simulink model "FixedwingModelR2020b"  (R2020b)
settings: Solver=ode4  StartTime=0.0  StopTime=100  FixedStep=0.001  RelTol=1e-3
PreLoadFcn:
  | filepath  = fileparts(get_param(bdroot, 'FileName'))
  | cd(filepath);
InitFcn:
  | Init
  | InitData
values from neighbouring files (symbols this model uses):
  env = struct    [InitData.m]
  ModelInit_Inputs = [0 0 -1 0 0 0 0 0 0 0 0 0 0 0 0 0]    [Init.m]
  ModelParam_envAltitude = -50    [Init.m]
  ModelParam_GPSEphFinal = 0.3    [Init.m]
  ModelParam_GPSEpvFinal = 0.4    [Init.m]
  ModelParam_noiseGPSSampTime = 0.2    [Init.m]
  ModelParam_noisePowerOffGainAccel = 0.04    [Init.m]
  ModelParam_noisePowerOffGainAccelZ = 0.03    [Init.m]
  ModelParam_noisePowerOffGainGyro = 0.02    [Init.m]
  ModelParam_noisePowerOffGainGyroZ = 0.025    [Init.m]
  ModelParam_noisePowerOffGainMag = 0.02    [Init.m]
  ModelParam_noisePowerOffGainMagZ = 0.035    [Init.m]
  ModelParam_noisePowerOnGainAccel = 0.8    [Init.m]
  ModelParam_noisePowerOnGainAccelZ = 4.5    [Init.m]
  ModelParam_noisePowerOnGainGyro = 2    [Init.m]
  ModelParam_noisePowerOnGainGyroZ = 1    [Init.m]
  ModelParam_noisePowerOnGainMag = 0.025    [Init.m]
  ModelParam_noisePowerOnGainMagZ = 0.05    [Init.m]
  ModelParam_uavType = int8(100)    [Init.m]
  uav = struct    [InitData.m]
undefined symbols (not defined in the file or in its folder): Earth, F, Light, MIL, ModelParam_GPSEpvInitial, ModelParam_GPSEpvTimeConstant, Newton, Raphson, WGS84
libraries: sharedtransform x6, aerolibactuator x5, FixedwingModelLib x4, aerolibasang x4, aerolibtransform2 x2, aerolibatmos2 x2, aerolibconvert2 x2, simulink x2, aerolibutil x2, aerolibwind2 x2, aerolibobsolete x1, shared6dof x1
(part 1 of 2)
settings Model: Creator=Jinrui  LastModifiedBy=dzl20201126
settings DataIOCC: ReturnWorkspaceOutputs=off
settings OptimizationCC: ZeroExternalMemoryAtStartup=off  ZeroInternalMemoryAtStartup=off  EfficientTunableParamExpr=on
settings DebuggingCC: ParameterTunabilityLossMsg=error  ArithmeticOperatorsInVariantConditions=warning
settings SFSimCC: SimUseLocalCustomCode=off  MATLABDynamicMemAlloc=off  CustomCodeUndefinedFunction=UseInterfaceOnly  SimTargetLang=C++
settings RTWCC: Description=Embedded Coder  SystemTargetFile=ert.tlc  GenCodeOnly=on  GenerateMakefile=off  PackageGeneratedCodeAndArtifacts=on  PackageName=MulticopterModel  TemplateMakefile=ert_default_tmf  RTWUseLocalCustomCode=off  TargetLang=C++  RTWCompilerOptimization=on
settings CodeAppCC: ForceParamTrailComments=on  OperatorAnnotations=on  SimulinkDataObjDesc=on  SFDataObjDesc=on  MATLABFcnDesc=on  InsertBlockDesc=on  StateflowObjectComments=on  MATLABSourceComments=on
settings ERTTargetCC: TargetLangStandard=C++03 (ISO)  MultiwordLength=2048  GenerateSampleERTMain=on  CodeInterfacePackaging=C++ class  SupportContinuousTime=on  MultiInstanceErrorCode=None  RootIOFormat=Structure reference  ERTCustomFileTemplate=example_file_process.tlc  ERTFilePackagingFormat=Compact
settings SimscapeCC: SimscapeNormalizeSystem=off

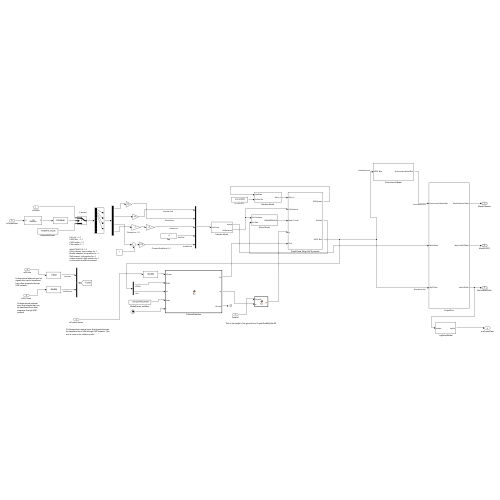
[thumbnail: Simulink's stored preview of the top-level diagram]
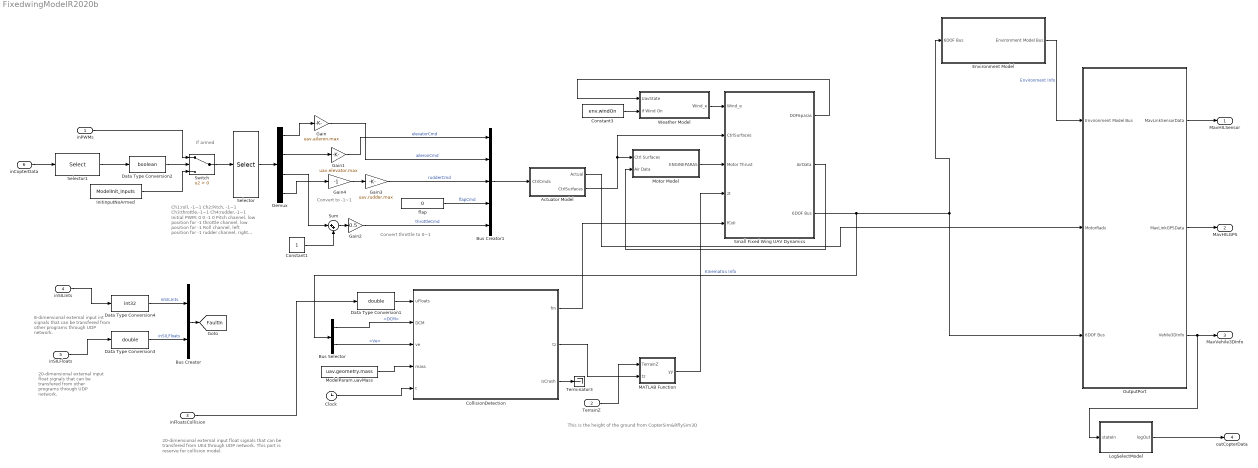
== system FixedwingModelR2020b ==
  note: Convert to -1~1
  note: Convert throttle to 0~1
  note: Ch1:roll, -1~1
      | Ch2:Pitch, -1~1
      | Ch3:throttle,-1~1
      | Ch4:rudder,-1~1
      |
      | Initial PWM: 0 0 -1 0
      | Pitch channel, low position for -1
      | throttle channel, low position for -1
      | Roll channel, left position for -1
      | rudder channel, right position for -1, so the value should be reversed
  note: This is the height of the ground from CopterSim&RflySim3D
  note: 20-dimensional external input float signals that can be transfered from UE4 through UDP network. This port is reserve for collision model.
  note: If armed
  note: 20-dimensional external input float signals that can be transfered from other programs through UDP network.
  note: 8-dimensional external input int signals that can be transfered from other programs through UDP network.
  inPWMs : Inport  PortDimensions=16
  TerrainZ : Inport  Port=2
  inFloatsCollision : Inport  Port=3  OutDataTypeStr=single  PortDimensions=20
  inSILInts : Inport  Port=4  OutDataTypeStr=int32  PortDimensions=8
  inSILFloats : Inport  Port=5  OutDataTypeStr=single  PortDimensions=20
  inCopterData : Inport  Port=6  OutDataTypeStr=double  PortDimensions=32
  Actuator Model : Subsystem
  Bus Creator : BusCreator  Inputs=2
  Bus Creator1 : BusCreator  Inputs=5
  Bus Selector : BusSelector  OutputSignals=DCM,Ve
  Clock : Clock
  CollisionDetection : MATLAB Function  TreatAsAtomicUnit=on
  Constant1 : Constant
  Constant3 : Constant  Value=env.windOn
      settings: AttributesFormatString=%<Value>
  Data Type Conversion1 : DataTypeConversion  OutDataTypeStr=double
  Data Type Conversion2 : DataTypeConversion  OutDataTypeStr=boolean
  Data Type Conversion3 : DataTypeConversion  OutDataTypeStr=double
  Data Type Conversion4 : DataTypeConversion  OutDataTypeStr=int32
  Demux : Demux
  Environment Model : Subsystem
  Gain : Gain  Gain=uav.aileron.max
  Gain1 : Gain  Gain=uav.elevator.max
  Gain2 : Gain  Gain=0.5
  Gain3 : Gain  Gain=uav.rudder.max
  Gain4 : Gain  Gain=-1
  InitinputNoArmed : Constant  Value=ModelInit_Inputs
  LogSelectModel : Subsystem
  MATLAB Function : MATLAB Function  TreatAsAtomicUnit=on
  ModelParam.uavMass : Constant  Value=uav.geometry.mass
  Motor Model : Subsystem
  OutputPort : Subsystem
  Selector : Selector  InputPortWidth=16  IndexOptions=Index vector (dialog)  Indices=[1 2 3 4]  OutputSizes=1
  Selector1 : Selector  InputPortWidth=32  IndexOptions=Index vector (dialog)  Indices=[1]  OutputSizes=1
  Small Fixed Wing UAV Dynamics : Subsystem
  Sum : Sum  Inputs=|++
  Switch : Switch  Criteria=u2 > Threshold
  Terminator3 : Terminator
  Weather Model : Subsystem
  flap : Constant  Value=0  OutDataTypeStr=double
  MavHILSensor : Outport  OutDataTypeStr=Bus: MavLinkSensor  VectorParamsAs1DForOutWhenUnconnected=off
  MavHILGPS : Outport  Port=2  OutDataTypeStr=Bus: MavLinkGPS  VectorParamsAs1DForOutWhenUnconnected=off
  MavVehile3DInfo : Outport  Port=3  OutDataTypeStr=Bus: MavVehileInfo  VectorParamsAs1DForOutWhenUnconnected=off
  outCopterData : Outport  Port=4  OutDataTypeStr=double  PortDimensions=32  VectorParamsAs1DForOutWhenUnconnected=off
  tag scope: FaultIn=global
  wires:
  Sum/1 -> Gain2/1
  Actuator Model/1(Actual) -> OutputPort/2(MotorRads)
  Demux/3 -> Sum/1
  Demux/1 -> Gain/1
  inPWMs/1 -> Switch/1
  Selector/1 -> Demux/1
  Demux/2 -> Gain1/1
  Small Fixed Wing UAV Dynamics/3(6DOF Bus) -> Bus Selector/1, Environment Model/1(6DOF Bus), OutputPort/3(6DOF Bus)  "Kinematics Info"
  Constant1/1 -> Sum/2
  Environment Model/1(Environment Model Bus) -> OutputPort/1(Environment Model Bus)  "Environment Info"
  Switch/1 -> Selector/1
  CollisionDetection/2(tz) -> MATLAB Function/2(tz)
  Actuator Model/2(CtrlSurfaces) -> Motor Model/1(Ctrl Surfaces), Small Fixed Wing UAV Dynamics/2(CtrlSurfaces)
  Small Fixed Wing UAV Dynamics/1(DOF6paras) -> Weather Model/1(UavState)
  Motor Model/1(ENGINEPARAS) -> Small Fixed Wing UAV Dynamics/3(Motor Thrust)
  Bus Creator1/1 -> Actuator Model/1(CtrlCmds)
  Constant3/1 -> Weather Model/2(if Wind On)
  Weather Model/1(Wind_e) -> Small Fixed Wing UAV Dynamics/1(Wind_e)
  Small Fixed Wing UAV Dynamics/2(AirData) -> Motor Model/2(Air Data)
  Gain3/1 -> Bus Creator1/3  "rudderCmd"
  flap/1 -> Bus Creator1/4  "flapCmd"
  Gain/1 -> Bus Creator1/2  "aileronCmd"
  Gain1/1 -> Bus Creator1/1  "elevatorCmd"
  Demux/4 -> Gain4/1
  Gain2/1 -> Bus Creator1/5  "throttleCmd"
  Gain4/1 -> Gain3/1
  CollisionDetection/1(fm) -> Small Fixed Wing UAV Dynamics/5(fColi)
  TerrainZ/1 -> MATLAB Function/1(TerrainZ)
  Bus Selector/1 -> CollisionDetection/2(DCM)  "<DCM>"
  Bus Selector/2 -> CollisionDetection/3(ve)  "<Ve>"
  ModelParam.uavMass/1 -> CollisionDetection/4(mass)
  Clock/1 -> CollisionDetection/5(t)
  Data Type Conversion1/1 -> CollisionDetection/1(uFloats)
  MATLAB Function/1(yy) -> Small Fixed Wing UAV Dynamics/4(zt)
  inFloatsCollision/1 -> Data Type Conversion1/1
  CollisionDetection/3(isCrash) -> Terminator3/1
  OutputPort/3(Vehile3DInfo) -> LogSelectModel/1(stateIn), MavVehile3DInfo/1
  OutputPort/2(MavLinkGPSData) -> MavHILGPS/1
  OutputPort/1(MavLinkSensorData) -> MavHILSensor/1
  Selector1/1 -> Data Type Conversion2/1
  inCopterData/1 -> Selector1/1
  InitinputNoArmed/1 -> Switch/3
  Data Type Conversion2/1 -> Switch/2
  Data Type Conversion3/1 -> Bus Creator/2  "inSILFloats"
  Bus Creator/1 -> [FaultIn]
  inSILFloats/1 -> Data Type Conversion3/1
  inSILInts/1 -> Data Type Conversion4/1
  Data Type Conversion4/1 -> Bus Creator/1  "inSILInts"
  LogSelectModel/1(logOut) -> outCopterData/1

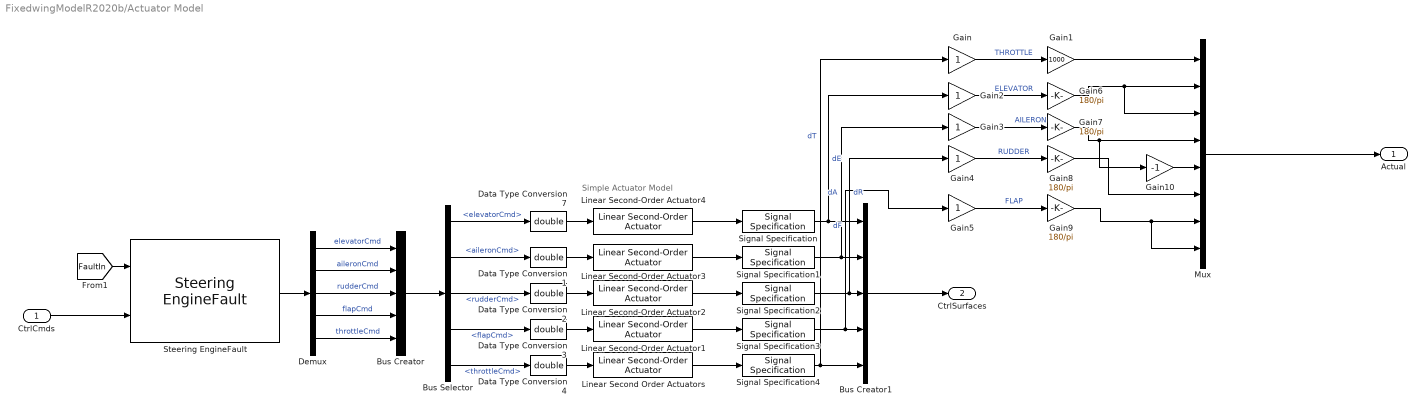
== system FixedwingModelR2020b/Actuator Model ==
  note: Simple Actuator Model
  CtrlCmds : Inport
  Bus Creator : BusCreator  Inputs=5
  Bus Creator1 : BusCreator  Inputs=5
  Bus Selector : BusSelector  OutputSignals=elevatorCmd,aileronCmd,rudderCmd,flapCmd,throttleCmd
  Data Type Conversion{1..4,7} (5 alike) : DataTypeConversion  OutDataTypeStr=double
  Demux : Demux  Outputs=5
  Gain{,2..5} (5 alike) : Gain
  Gain1 : Gain  Gain=1000
  Gain10 : Gain  Gain=-1
  Gain{6..9} (4 alike) : Gain  Gain=180/pi
  Linear Second Order Actuators : aerolibactuator/Linear Second-Order Actuator  wn_fin=35  z_fin=0.75  fin_act_0=0  fin_act_vel=0
      settings: SourceProductBaseCode=AE
      settings: AttributesFormatString=|
      | Nat Freq => %<wn_fin>
      | Damping => %<z_fin>
  Linear Second-Order Actuator{1..4} (4 alike) : aerolibactuator/Linear Second-Order Actuator  wn_fin=35  z_fin=0.75  fin_act_0=0  fin_act_vel=0
      settings: SourceProductBaseCode=AE
  Mux : Mux  Inputs=8
  Signal Specification{,1..3} (4 alike) : SignalSpecification  Unit=rad
  Signal Specification4 : SignalSpecification  Unit=%
  Steering EngineFault : FixedwingModelLib/Steering EngineFault  FaultParamStruct=SteerEngineFault  ComParamVect=FaultParamAPI
  Actual : Outport  VectorParamsAs1DForOutWhenUnconnected=off
  CtrlSurfaces : Outport  Port=2  VectorParamsAs1DForOutWhenUnconnected=off
  wires:
  Data Type Conversion7/1 -> Linear Second-Order Actuator4/1
  Data Type Conversion1/1 -> Linear Second-Order Actuator3/1
  Data Type Conversion2/1 -> Linear Second-Order Actuator2/1
  Data Type Conversion3/1 -> Linear Second-Order Actuator1/1
  Data Type Conversion4/1 -> Linear Second Order Actuators/1
  Bus Selector/1 -> Data Type Conversion7/1  "<elevatorCmd>"
  Linear Second-Order Actuator2/1 -> Signal Specification2/1
  Linear Second-Order Actuator3/1 -> Signal Specification1/1
  Linear Second-Order Actuator1/1 -> Signal Specification3/1
  Linear Second-Order Actuator4/1 -> Signal Specification/1
  Bus Selector/4 -> Data Type Conversion3/1  "<flapCmd>"
  Bus Selector/5 -> Data Type Conversion4/1  "<throttleCmd>"
  Bus Selector/3 -> Data Type Conversion2/1  "<rudderCmd>"
  Bus Selector/2 -> Data Type Conversion1/1  "<aileronCmd>"
  Linear Second Order Actuators/1 -> Signal Specification4/1
  Signal Specification/1 -> Gain2/1, Bus Creator1/1  "dE"
  Signal Specification1/1 -> Gain3/1, Bus Creator1/2  "dA"
  Signal Specification2/1 -> Gain4/1, Bus Creator1/3  "dR"
  Signal Specification4/1 -> Gain/1, Bus Creator1/5  "dT"
  Gain1/1 -> Mux/1
  Gain/1 -> Gain1/1  "THROTTLE"
  Gain2/1 -> Gain6/1  "ELEVATOR"
  Gain4/1 -> Gain8/1  "RUDDER"
  Gain3/1 -> Gain7/1  "AILERON"
  Signal Specification3/1 -> Gain5/1, Bus Creator1/4  "dF"
  Gain5/1 -> Gain9/1  "FLAP"
  Gain6/1 -> Mux/3, Mux/2
  Gain7/1 -> Gain10/1, Mux/4
  Gain8/1 -> Mux/6
  Gain9/1 -> Mux/8, Mux/7
  Gain10/1 -> Mux/5
  Mux/1 -> Actual/1
  Bus Creator1/1 -> CtrlSurfaces/1
  Demux/3 -> Bus Creator/3  "rudderCmd"
  Demux/5 -> Bus Creator/5  "throttleCmd"
  Demux/1 -> Bus Creator/1  "elevatorCmd"
  [FaultIn] -> Steering EngineFault/1
  Demux/4 -> Bus Creator/4  "flapCmd"
  Steering EngineFault/1 -> Demux/1
  Demux/2 -> Bus Creator/2  "aileronCmd"
  CtrlCmds/1 -> Steering EngineFault/2
  Bus Creator/1 -> Bus Selector/1

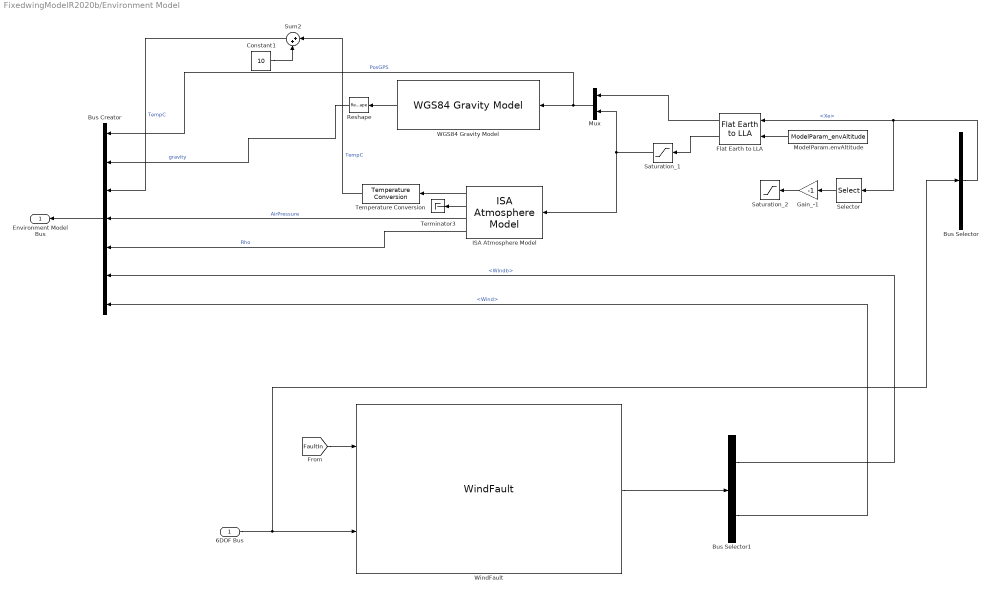
== system FixedwingModelR2020b/Environment Model ==
  6DOF Bus : Inport
  Bus Creator : BusCreator  Inputs=7
  Bus Selector : BusSelector  OutputSignals=Xe
  Bus Selector1 : BusSelector  OutputSignals=Windb,Wind
  Constant1 : Constant  Value=10
  Flat Earth to LLA : aerolibtransform2/Flat Earth to LLA  units=Metric (MKS)  ptype=Earth (WGS84)  F=1/298.257223563  R=6378137  refPosPort=off  LL0=ModelParam_GPSLatLong  psi=0
  Gain_-1 : Gain  Gain=-1
  ISA Atmosphere Model : aerolibatmos2/ISA Atmosphere Model  custom=off  g=9.80665  gamma=1.4  R=287.0531  L=0.0065  h_trop=11000  h_strat=20000  rho0=1.225  P0=101325  T0=288.15  h0=0
  ModelParam.envAltitude : Constant  Value=ModelParam_envAltitude
  Mux : Mux  Inputs=2
  Reshape : Reshape
  Saturation_1 : Saturate  UpperLimit=100000  LowerLimit=0
  Saturation_2 : Saturate  UpperLimit=10000  LowerLimit=0
  Selector : Selector  InputPortWidth=3  IndexOptions=Index vector (dialog)  Indices=[3]  OutputSizes=1
  Sum2 : Sum  Inputs=|++
  Temperature Conversion : aerolibconvert2/Temperature Conversion  IU=K  OU=C
      settings: SourceProductBaseCode=AE
  Terminator3 : Terminator
  "WGS84 Gravity Model " : aerolibobsolete/WGS84 Gravity Model   model=WGS84 Taylor Series  units=Metric (MKS)  no_atmos=on  precessing=on  jd_loc=off  month=October  day=10  year=2004  no_centrifugal=on  action=Warning
      settings: SourceProductBaseCode=AE
  WindFault : FixedwingModelLib/WindFault  FaultParamStruct=WindFault  ComParamVect=FaultParamAPI
  Environment Model Bus : Outport  VectorParamsAs1DForOutWhenUnconnected=off
  wires:
  ISA Atmosphere Model/4 -> Bus Creator/5  "Rho"
  [FaultIn] -> WindFault/1
  6DOF Bus/1 -> WindFault/2, Bus Selector/1
  Flat Earth to LLA/2 -> Saturation_1/1
  WindFault/1 -> Bus Selector1/1
  Sum2/1 -> Bus Creator/3  "TempC"
  ModelParam.envAltitude/1 -> Flat Earth to LLA/2
  Gain_-1/1 -> Saturation_2/1
  Bus Selector1/1 -> Bus Creator/6  "<Windb>"
  Saturation_1/1 -> Mux/2, ISA Atmosphere Model/1
  ISA Atmosphere Model/1 -> Temperature Conversion/1
  "WGS84 Gravity Model "/1 -> Reshape/1
  Bus Selector1/2 -> Bus Creator/7  "<Wind>"
  Bus Creator/1 -> Environment Model Bus/1
  Bus Selector/1 -> Selector/1, Flat Earth to LLA/1  "<Xe>"
  Temperature Conversion/1 -> Sum2/1  "TempC"
  Mux/1 -> Bus Creator/1, "WGS84 Gravity Model "/1  "PosGPS"
  Selector/1 -> Gain_-1/1
  ISA Atmosphere Model/3 -> Bus Creator/4  "AirPressure"
  Flat Earth to LLA/1 -> Mux/1
  ISA Atmosphere Model/2 -> Terminator3/1
  Reshape/1 -> Bus Creator/2  "gravity"
  Constant1/1 -> Sum2/2

== system FixedwingModelR2020b/LogSelectModel ==
  note: 1:3
  note: 4:6
  note: 7:9
  stateIn : Inport
  Bus Selector : BusSelector  OutputSignals=AccB,RateB,VelE
  Bus Selector1 : BusSelector  OutputSignals=PWM
  Constant : Constant  Value=[0,0,0,0,0,0,0,0,0,0,0,0,0,0,0,0,0,0]
  Data Type Conversion{,1..3} (4 alike) : DataTypeConversion  OutDataTypeStr=double
  Mux12 : Mux  Inputs=5
  logOut : Outport
  wires:
  stateIn/1 -> Bus Selector/1
  Bus Selector/1 -> Data Type Conversion/1  "<AccB>"
  Bus Selector/2 -> Data Type Conversion1/1  "<RateB>"
  Bus Selector/3 -> Data Type Conversion2/1  "<VelE>"
  [is123450] -> Bus Selector1/1
  Bus Selector1/1 -> Data Type Conversion3/1  "<PWM>"
  Data Type Conversion/1 -> Mux12/1
  Data Type Conversion1/1 -> Mux12/2
  Data Type Conversion2/1 -> Mux12/3
  Data Type Conversion3/1 -> Mux12/4
  Mux12/1 -> logOut/1
  Constant/1 -> Mux12/5

== system FixedwingModelR2020b/Motor Model ==
  Ctrl Surfaces : Inport
  Air Data : Inport  Port=2
  Bus Creator1 : BusCreator  Inputs=6
  Bus Selector : BusSelector  OutputSignals=dT
  Bus Selector1 : BusSelector  OutputSignals=airpseed
  Constant{1..5} (5 alike) : Constant  Value=0
  Engine Model : Subsystem
  ENGINEPARAS : Outport  VectorParamsAs1DForOutWhenUnconnected=off
  wires:
  Bus Selector1/1 -> Engine Model/2(Airspeed)  "<airpseed>"
  Ctrl Surfaces/1 -> Bus Selector/1
  Air Data/1 -> Bus Selector1/1
  Bus Selector/1 -> Engine Model/1(dt)  "<dT>"
  Engine Model/1(Thrust_b) -> Bus Creator1/1  "Fx_eng"
  Constant4/1 -> Bus Creator1/5  "M_eng"
  Constant3/1 -> Bus Creator1/4  "R_eng"
  Constant5/1 -> Bus Creator1/6  "N_eng"
  Constant2/1 -> Bus Creator1/3  "Fz_eng"
  Constant1/1 -> Bus Creator1/2  "Fy_eng"
  Bus Creator1/1 -> ENGINEPARAS/1

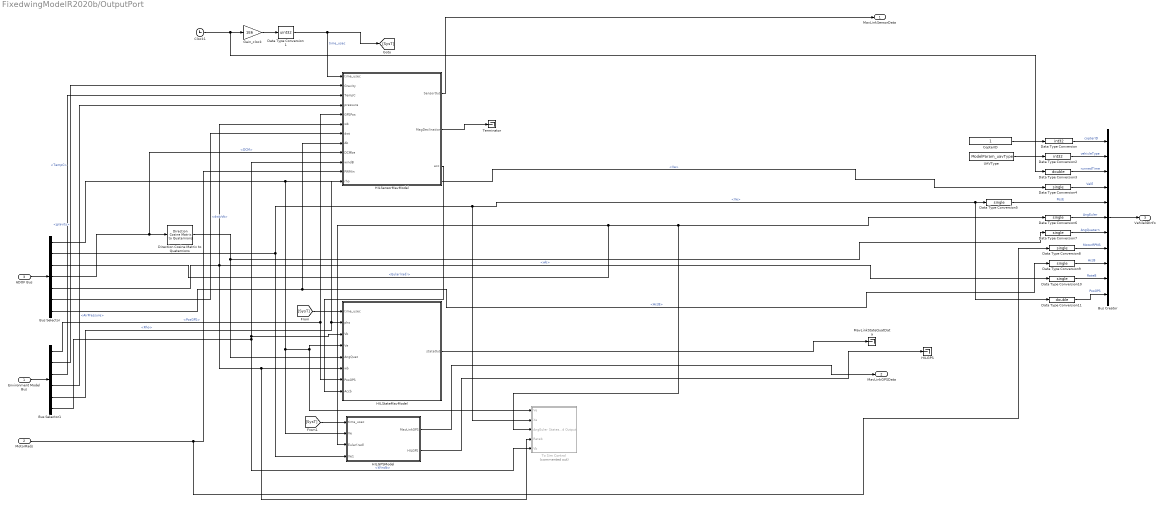
== system FixedwingModelR2020b/OutputPort ==
  Environment Model Bus : Inport
  MotorRads : Inport  Port=2
  6DOF Bus : Inport  Port=3
  Bus Creator : BusCreator  Inputs=11  OutDataTypeStr=Bus: MavVehileInfo
  Bus Selector : BusSelector  OutputSignals=Ve,Xe,Eular(rad),DCM,wb,dwb/dt,AccB
  Bus Selector1 : BusSelector  OutputSignals=PosGPS,gravity,TempC,AirPressure,Rho,Windb
  Clock1 : Clock
  CopterID : Constant
  Data Type Conversion : DataTypeConversion  OutDataTypeStr=int32
  Data Type Conversion1 : DataTypeConversion  OutDataTypeStr=uint32
  Data Type Conversion{4..10} (7 alike) : DataTypeConversion  OutDataTypeStr=single
  Data Type Conversion11 : DataTypeConversion  OutDataTypeStr=double
  Data Type Conversion2 : DataTypeConversion  OutDataTypeStr=int32
  Data Type Conversion3 : DataTypeConversion  OutDataTypeStr=double
  Direction Cosine Matrix to Quaternions : sharedtransform/Direction Cosine Matrix  to Quaternions  aMode=aMode  action=None  tolerance=eps(2)
      settings: SourceProductBaseCode=AE,PW,DR,MT,VE
  Gain_clock : Gain  Gain=1E6
  HILGPS : Terminator
  HILGPSModel : Subsystem
  HILSensorMavModel : Subsystem
  HILStateMavModel : Subsystem
  MavLinkStateQuatData : Terminator
  Terminator : Terminator
  To Sim Control : Subsystem  Commented=on
  UAVType : Constant  Value=ModelParam_uavType
  MavLinkSensorData : Outport  VectorParamsAs1DForOutWhenUnconnected=off
  MavLinkGPSData : Outport  Port=2  VectorParamsAs1DForOutWhenUnconnected=off
  Vehile3DInfo : Outport  Port=3  VectorParamsAs1DForOutWhenUnconnected=off
  wires:
  [SysT] -> HILGPSModel/1(time_usec)
  [SysT] -> HILStateMavModel/1(time_usec)
  Bus Selector/5 -> HILSensorMavModel/6(wb), Data Type Conversion10/1, HILStateMavModel/6(wb), To Sim Control/4(Rateb)  "<wb>"
  Bus Selector/4 -> HILSensorMavModel/9(DCMbe), Direction Cosine Matrix to Quaternions/1  "<DCM>"
  Bus Selector/1 -> HILGPSModel/2(Ve), HILStateMavModel/4(Ve), To Sim Control/1(Ve), Data Type Conversion4/1  "<Ve>"
  Bus Selector/6 -> HILSensorMavModel/7(dwt)  "<dwb/dt>"
  Bus Selector/3 -> Data Type Conversion6/1, To Sim Control/3(AngEuler), HILGPSModel/3(Eular(rad))  "<Eular(rad)>"
  Clock1/1 -> Data Type Conversion3/1, Gain_clock/1
  Data Type Conversion1/1 -> HILSensorMavModel/1(time_usec), [SysT]  "time_usec"
  Gain_clock/1 -> Data Type Conversion1/1
  6DOF Bus/1 -> Bus Selector/1
  Environment Model Bus/1 -> Bus Selector1/1
  Bus Selector1/1 -> HILSensorMavModel/5(GPSPos), HILStateMavModel/7(PosGPS)  "<PosGPS>"
  Bus Selector1/2 -> HILSensorMavModel/2(Gravity)  "<gravity>"
  Bus Selector1/3 -> HILSensorMavModel/3(TempC)  "<TempC>"
  Bus Selector1/4 -> HILSensorMavModel/4(pressure)  "<AirPressure>"
  Bus Selector1/5 -> HILSensorMavModel/12(rho), HILStateMavModel/2(pho)  "<Rho>"
  Bus Selector1/6 -> HILSensorMavModel/10(windB), HILStateMavModel/3(Vb), To Sim Control/5(Vb)  "<Windb>"
  HILSensorMavModel/1(SensorOut) -> MavLinkSensorData/1
  Direction Cosine Matrix to Quaternions/1 -> HILStateMavModel/5(AngQuat), Data Type Conversion7/1
  HILStateMavModel/1(stateOut) -> MavLinkStateQuatData/1
  HILGPSModel/1(MavLinkGPS) -> MavLinkGPSData/1
  MotorRads/1 -> HILSensorMavModel/11(PWMin), Data Type Conversion8/1
  Bus Selector/7 -> HILSensorMavModel/8(Ab), Data Type Conversion9/1  "<AccB>"
  CopterID/1 -> Data Type Conversion/1
  Data Type Conversion/1 -> Bus Creator/1  "copterID"
  Data Type Conversion2/1 -> Bus Creator/2  "vehicleType"
  UAVType/1 -> Data Type Conversion2/1
  Data Type Conversion3/1 -> Bus Creator/3  "runnedTime"
  Data Type Conversion4/1 -> Bus Creator/4  "VelE"
  Data Type Conversion5/1 -> Bus Creator/5  "PosE"
  Data Type Conversion6/1 -> Bus Creator/6  "AngEuler"
  Data Type Conversion7/1 -> Bus Creator/7  "AngQuatern"
  Data Type Conversion8/1 -> Bus Creator/8  "MotorRPMS"
  Data Type Conversion9/1 -> Bus Creator/9  "AccB"
  Data Type Conversion10/1 -> Bus Creator/10  "RateB"
  Data Type Conversion11/1 -> Bus Creator/11  "PosGPS"
  Bus Creator/1 -> Vehile3DInfo/1
  Bus Selector/2 -> HILGPSModel/4(Xe1), Data Type Conversion11/1, Data Type Conversion5/1, To Sim Control/2(Xe)  "<Xe>"
  HILSensorMavModel/2(MagDeclination) -> Terminator/1
  HILSensorMavModel/3(acc) -> HILStateMavModel/8(Accb)
  HILGPSModel/2(HILGPS) -> HILGPS/1

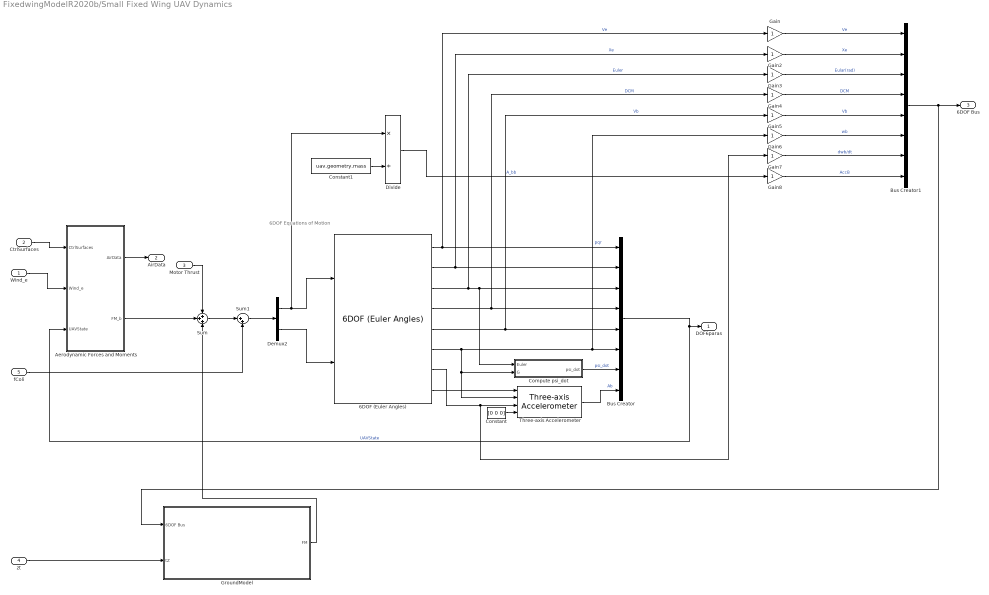
== system FixedwingModelR2020b/Small Fixed Wing UAV Dynamics ==
  note: 6DOF Equations of Motion
  Wind_e : Inport
  CtrlSurfaces : Inport  Port=2
  Motor Thrust : Inport  Port=3
  zt : Inport  Port=4
  fColi : Inport  Port=5
  6DOF (Euler Angles) : shared6dof/6DOF (Euler Angles)  units=Metric (MKS)  mtype=Fixed  rep=Euler Angles  xme_0=ModelInit_PosE  Vm_0=ModelInit_VelB  eul_0=ModelInit_AngEuler  pm_0=ModelInit_RateB  mass_0=uav.geometry.mass  mass_e=0.5  mass_f=2.0  inertia=eye(3).*[uav.inertia.Ixx;uav.inertia.Iyy; uav.inertia.Izz]  inertia_e=eye(3)  inertia_f=2*eye(3)  k_quat=1.0  vre_flag=on  abi_flag=off  aMode=aMode  xme_statename=''  Vm_statename=''  eul_statename=''  quat_statename=''  pm_statename=''  mass_statename=''
      settings: SourceProductBaseCode=AE,PW,DR,MT,VE
  Aerodynamic Forces and Moments : Subsystem
  Bus Creator : BusCreator  Inputs=8
  Bus Creator1 : BusCreator  Inputs=8
  Compute psi_dot : Subsystem
  Constant : Constant  Value=[0 0 0]
      settings: AttributesFormatString=%<Value>
  Constant1 : Constant  Value=uav.geometry.mass
  Demux2 : Demux  Outputs=2
  Divide : Product  Inputs=*/
  Gain{,2..8} (8 alike) : Gain
  GroundModel : Subsystem
  Sum : Sum  Inputs=+++  SaturateOnIntegerOverflow=on
  Sum1 : Sum  Inputs=|++
  Three-axis Accelerometer : aerolibnav/Three-axis Accelerometer  units=Metric (MKS)  acc=[0 0 0]  gtype=off  dtype_a=off  w_a=190  z_a=0.707  a_sf_cc=[1 0 0; 0 1 0; 0 0 1]  a_bias=[0 0 0]  a_Ts=0  a_rand=off  a_seeds=[23093 23094 23095]  a_pow=[0.001 0.001 0.001]  a_sat="[-inf  -inf  -inf  inf inf inf]"
      settings: SourceProductBaseCode=AE
  DOF6paras : Outport  VectorParamsAs1DForOutWhenUnconnected=off
  AirData : Outport  Port=2  VectorParamsAs1DForOutWhenUnconnected=off
  6DOF Bus : Outport  Port=3  VectorParamsAs1DForOutWhenUnconnected=off
  wires:
  Motor Thrust/1 -> Sum/1
  Aerodynamic Forces and Moments/1(AirData) -> AirData/1
  Aerodynamic Forces and Moments/2(FM_b) -> Sum/2
  Wind_e/1 -> Aerodynamic Forces and Moments/2(Wind_e)
  CtrlSurfaces/1 -> Aerodynamic Forces and Moments/1(CtrlSurfaces)
  Sum/1 -> Sum1/1
  Demux2/2 -> 6DOF (Euler Angles)/2
  Constant/1 -> Three-axis Accelerometer/4
  Bus Creator/1 -> DOF6paras/1, Aerodynamic Forces and Moments/3(UAVState)  "UAVState"
  Three-axis Accelerometer/1 -> Bus Creator/8  "Ab"
  6DOF (Euler Angles)/8 -> Three-axis Accelerometer/1
  6DOF (Euler Angles)/3 -> Gain3/1, Bus Creator/3, Compute psi_dot/1(Euler)  "Euler"
  6DOF (Euler Angles)/1 -> Gain/1, Bus Creator/1  "Ve"
  Compute psi_dot/1(psi_dot) -> Bus Creator/7  "psi_dot"
  6DOF (Euler Angles)/4 -> Gain4/1, Bus Creator/4  "DCM"
  6DOF (Euler Angles)/5 -> Gain5/1, Bus Creator/5  "Vb"
  6DOF (Euler Angles)/2 -> Gain2/1, Bus Creator/2  "Xe"
  6DOF (Euler Angles)/6 -> Three-axis Accelerometer/2, Compute psi_dot/2(G), Gain6/1, Bus Creator/6  "pqr"
  6DOF (Euler Angles)/7 -> Gain7/1, Three-axis Accelerometer/3
  Gain6/1 -> Bus Creator1/6  "wb"
  Gain2/1 -> Bus Creator1/2  "Xe"
  Gain/1 -> Bus Creator1/1  "Ve"
  Gain7/1 -> Bus Creator1/7  "dwb/dt"
  Gain5/1 -> Bus Creator1/5  "Vb"
  Gain4/1 -> Bus Creator1/4  "DCM"
  Bus Creator1/1 -> GroundModel/1(6DOF Bus), 6DOF Bus/1
  Gain8/1 -> Bus Creator1/8  "AccB"
  Gain3/1 -> Bus Creator1/3  "Eular(rad)"
  Demux2/1 -> Divide/1, 6DOF (Euler Angles)/1
  Divide/1 -> Gain8/1  "A_bb"
  Constant1/1 -> Divide/2
  zt/1 -> GroundModel/2("tZ ")
  GroundModel/1(FM) -> Sum/3
  fColi/1 -> Sum1/2
  Sum1/1 -> Demux2/1

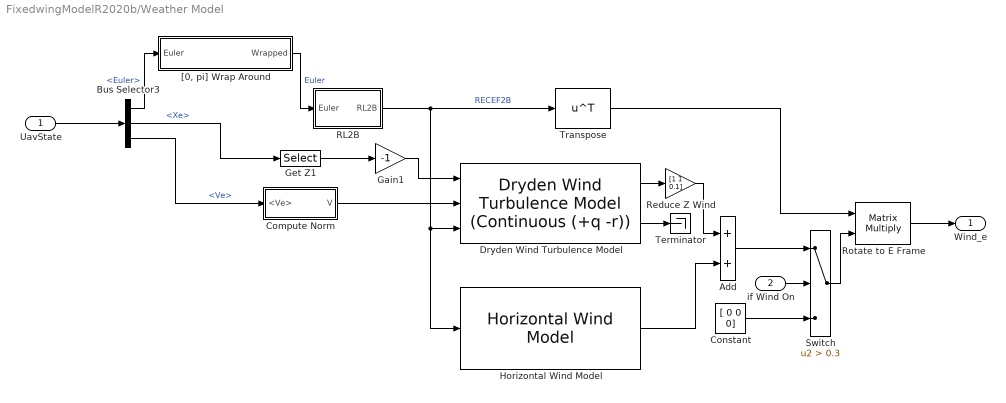
== system FixedwingModelR2020b/Weather Model ==
  UavState : Inport
  if Wind On : Inport  Port=2
  " Compute Norm" : Subsystem
  Add : Sum  Inputs=2
  Bus Selector3 : BusSelector  OutputSignals=Euler,Xe,Ve
  Constant : Constant  Value=[ 0 0 0]
      settings: AttributesFormatString=%<Value>
  Dryden Wind Turbulence Model : aerolibwind2/Dryden Wind Turbulence Model  (Continuous (+q -r))  units=Metric (MKS)  spec=MIL-F-8785C  model=Continuous Dryden (+q -r)  W20=env.windBase/4  Wdeg=env.windDirTurb  TurbProb=10^-2 - Light  L_high=533.4  Wingspan=uav.geometry.span  ts=ap.apSampleTime  Seed=[23341 23342 23343 23344]  T_on=on
  Gain1 : Gain  Gain=-1
      settings: AttributesFormatString=Z to Alt
  Get Z1 : Selector  InputPortWidth=3  IndexOptions=Index vector (dialog)  Indices=[3]  OutputSizes=[(-2)]
  "Horizontal Wind Model " : aerolibwind2/Horizontal Wind Model  units=Metric (MKS)  Vw_source=Internal  Vwind=env.windBase  W_source=Internal  Wdeg=env.windDirHor
      settings: SourceProductBaseCode=AE
  RL2B : Subsystem
  Reduce Z Wind : Gain  Gain=[1 1 0.1]
      settings: AttributesFormatString=%<Gain>
  Rotate to E Frame : Product  Multiplication=Matrix(*)
  Switch : Switch  Criteria=u2 > Threshold  Threshold=0.3
  Terminator : Terminator
  Transpose : Math  Operator=transpose  SignedPower=on  SaturateOnIntegerOverflow=on
  "[0, pi] Wrap Around" : Subsystem
  Wind_e : Outport  Unit=m/s  VectorParamsAs1DForOutWhenUnconnected=off
  wires:
  Bus Selector3/2 -> Get Z1/1  "<Xe>"
  Bus Selector3/1 -> "[0, pi] Wrap Around"/1(Euler)  "<Euler>"
  Dryden Wind Turbulence Model/2 -> Terminator/1
  Constant/1 -> Switch/3
  Get Z1/1 -> Gain1/1
  Bus Selector3/3 -> " Compute Norm"/1(<Ve>)  "<Ve>"
  RL2B/1(RL2B) -> Dryden Wind Turbulence Model/3, "Horizontal Wind Model "/1, Transpose/1  "RECEF2B"
  Transpose/1 -> Rotate to E Frame/1
  Rotate to E Frame/1 -> Wind_e/1
  Switch/1 -> Rotate to E Frame/2
  Dryden Wind Turbulence Model/1 -> Reduce Z Wind/1
  " Compute Norm"/1(V) -> Dryden Wind Turbulence Model/2
  UavState/1 -> Bus Selector3/1
  Gain1/1 -> Dryden Wind Turbulence Model/1
  "Horizontal Wind Model "/1 -> Add/2
  Reduce Z Wind/1 -> Add/1
  Add/1 -> Switch/1
  if Wind On/1 -> Switch/2
  "[0, pi] Wrap Around"/1(Wrapped) -> RL2B/1(Euler)  "Euler"

== system FixedwingModelR2020b/Motor Model/Engine Model ==
  dt : Inport
  Airspeed : Inport  Port=2
  Get To : Subsystem
  Mass Conversion : aerolibconvert2/Mass Conversion  IU=lbm  OU=kg
      settings: SourceProductBaseCode=AE
  Mux : Mux  Inputs=2
  Thrust Available (lbs) : Fcn  Expr=u(1) - 0.047*sqrt(u(1))*u(2)
  kg2N : Gain  Gain=env.ISA_g  SaturateOnIntegerOverflow=on  OutDataTypeStr=Inherit: Same as input  ParamDataTypeStr=Inherit: Same as input
      settings: AttributesFormatString=%<Gain>
  Thrust_b : Outport  Unit=kg*m/s^2  VectorParamsAs1DForOutWhenUnconnected=off
  wires:
  Mass Conversion/1 -> kg2N/1
  kg2N/1 -> Thrust_b/1
  Airspeed/1 -> Mux/2
  Thrust Available (lbs)/1 -> Mass Conversion/1
  Mux/1 -> Thrust Available (lbs)/1
  Get To/1(To) -> Mux/1
  dt/1 -> Get To/1(dt)

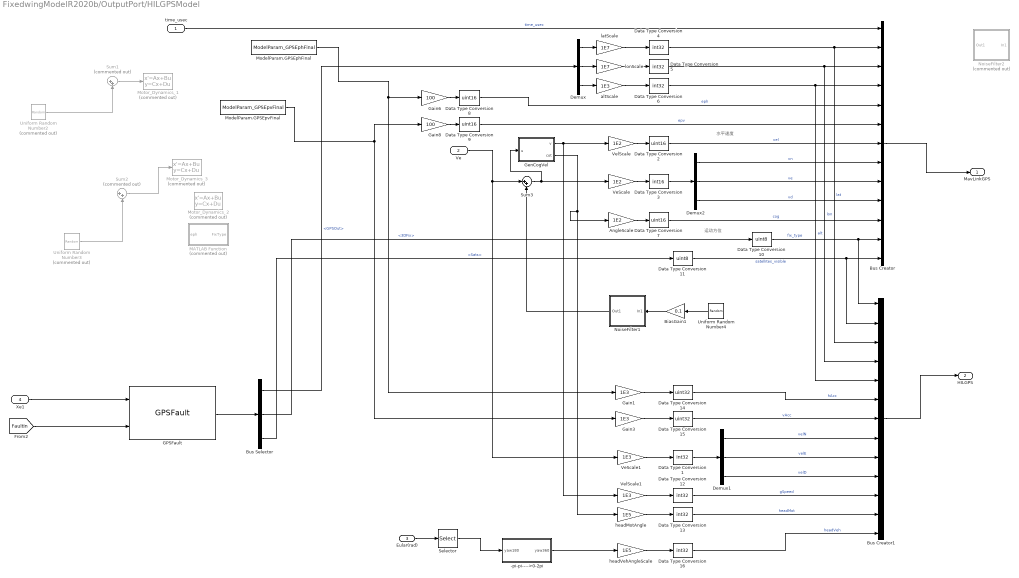
== system FixedwingModelR2020b/OutputPort/HILGPSModel ==
  note: 水平速度
  note: 运动方位
  time_usec : Inport
  Ve : Inport  Port=2
  Eular(rad) : Inport  Port=3
  Xe1 : Inport  Port=4
  -pi-pi---->0-2pi : MATLAB Function  TreatAsAtomicUnit=on
  AngleScale : Gain  Gain=1E2
  BiasGain1 : Gain  Gain=0.1
  Bus Creator : BusCreator  Inputs=13  OutDataTypeStr=Bus: MavLinkGPS  NonVirtualBus=on
  Bus Creator1 : BusCreator  Inputs=13  OutDataTypeStr=Bus: HILGPS  NonVirtualBus=on
  Bus Selector : BusSelector  OutputSignals=GPSOut,3DFix,Sats
  Data Type Conversion{1,4..6,12..13,16} (7 alike) : DataTypeConversion  OutDataTypeStr=int32  RndMeth=Round
  Data Type Conversion10 : DataTypeConversion  OutDataTypeStr=uint8  RndMeth=Round
  Data Type Conversion11 : DataTypeConversion  OutDataTypeStr=uint8  RndMeth=Round
  Data Type Conversion14 : DataTypeConversion  OutDataTypeStr=uint32  RndMeth=Round
  Data Type Conversion15 : DataTypeConversion  OutDataTypeStr=uint32  RndMeth=Round
  Data Type Conversion{2,7..9} (4 alike) : DataTypeConversion  OutDataTypeStr=uint16  RndMeth=Round
  Data Type Conversion3 : DataTypeConversion  OutDataTypeStr=int16  RndMeth=Round
  Demux : Demux  Outputs=3
  Demux1 : Demux  Outputs=3
  Demux2 : Demux  Outputs=3
  GPSFault : FixedwingModelLib/GPSFault  FaultParamStruct=SensorFault
  Gain1 : Gain  Gain=1E3
  Gain3 : Gain  Gain=1E3
  Gain6 : Gain  Gain=100
  Gain8 : Gain  Gain=100
  GenCogVel : MATLAB Function  TreatAsAtomicUnit=on
  MATLAB Function : MATLAB Function  Commented=on  TreatAsAtomicUnit=on
  ModelParam.GPSEphFinal : Constant  Value=ModelParam_GPSEphFinal
  ModelParam.GPSEpvFinal : Constant  Value=ModelParam_GPSEpvFinal
  Motor_Dynamics_1 : StateSpace  Commented=on  A=-1/0.2  C=1/0.2  D=0  InitialCondition=20*0.2
  Motor_Dynamics_2 : StateSpace  Commented=on  A=-1/ModelParam_GPSEpvTimeConstant  C=1/ModelParam_GPSEpvTimeConstant  D=0  InitialCondition=ModelParam_GPSEpvInitial*ModelParam_GPSEpvTimeConstant
  Motor_Dynamics_3 : StateSpace  Commented=on  A=-1/0.2  C=1/0.2  D=0  InitialCondition=20*0.2
  NoiseFilter1 : Subsystem
  NoiseFilter2 : Subsystem  Commented=on
  Selector : Selector  InputPortWidth=3  IndexOptions=Index vector (dialog)  Indices=[3]  OutputSizes=1
  Sum1 : Sum  Commented=on  Inputs=|++
  Sum2 : Sum  Commented=on  Inputs=|++
  Sum3 : Sum  Inputs=|++
  Uniform Random Number2 : UniformRandomNumber  Commented=on  Minimum=-0.01  Maximum=0.01  Seed=4345454  SampleTime=ModelParam_noiseGPSSampTime
  Uniform Random Number3 : UniformRandomNumber  Commented=on  Seed=3244333  SampleTime=ModelParam_noiseGPSSampTime
  Uniform Random Number4 : UniformRandomNumber  Minimum=[-1,-1,-2]  Maximum=[1,1,2]  Seed=[5445,45433,33433]  SampleTime=ModelParam_noiseGPSSampTime
  VeScale : Gain  Gain=1E2
  VeScale1 : Gain  Gain=1E3
  VelScale : Gain  Gain=1E2
  VelScale1 : Gain  Gain=1E3
  altScale : Gain  Gain=1E3
  headMotAngle : Gain  Gain=1E5
  headVehAngleScale : Gain  Gain=1E5
  latScale : Gain  Gain=1E7
  lonScale : Gain  Gain=1E7
  MavLinkGPS : Outport  VectorParamsAs1DForOutWhenUnconnected=off
  HILGPS : Outport  Port=2  VectorParamsAs1DForOutWhenUnconnected=off
  wires:
  Data Type Conversion16/1 -> Bus Creator1/13  "headVeh"
  headVehAngleScale/1 -> Data Type Conversion16/1
  Data Type Conversion13/1 -> Bus Creator1/12  "headMot"
  Data Type Conversion12/1 -> Bus Creator1/11  "gSpeed"
  Demux1/3 -> Bus Creator1/10  "velD"
  Demux1/2 -> Bus Creator1/9  "velE"
  Demux1/1 -> Bus Creator1/8  "velN"
  Data Type Conversion1/1 -> Demux1/1
  headMotAngle/1 -> Data Type Conversion13/1
  Data Type Conversion15/1 -> Bus Creator1/7  "vAcc"
  Data Type Conversion14/1 -> Bus Creator1/6  "hAcc"
  Gain3/1 -> Data Type Conversion15/1
  Gain1/1 -> Data Type Conversion14/1
  VeScale1/1 -> Data Type Conversion1/1
  VelScale1/1 -> Data Type Conversion12/1
  Data Type Conversion8/1 -> Bus Creator/5  "eph"
  Gain8/1 -> Data Type Conversion9/1
  Gain6/1 -> Data Type Conversion8/1
  Data Type Conversion9/1 -> Bus Creator/6  "epv"
  time_usec/1 -> Bus Creator/1  "time_usec"
  latScale/1 -> Data Type Conversion4/1
  lonScale/1 -> Data Type Conversion5/1
  altScale/1 -> Data Type Conversion6/1
  Data Type Conversion4/1 -> Bus Creator/2, Bus Creator1/3  "lat"
  Data Type Conversion5/1 -> Bus Creator/3, Bus Creator1/4  "lon"
  Data Type Conversion6/1 -> Bus Creator/4, Bus Creator1/5  "alt"
  Demux2/1 -> Bus Creator/8  "vn"
  Demux2/2 -> Bus Creator/9  "ve"
  Demux2/3 -> Bus Creator/10  "vd"
  VeScale/1 -> Data Type Conversion3/1
  Data Type Conversion3/1 -> Demux2/1
  VelScale/1 -> Data Type Conversion2/1
  Data Type Conversion2/1 -> Bus Creator/7  "vel"
  AngleScale/1 -> Data Type Conversion7/1
  Data Type Conversion7/1 -> Bus Creator/11  "cog"
  Data Type Conversion11/1 -> Bus Creator/13, Bus Creator1/2  "satellites_visible"
  Data Type Conversion10/1 -> Bus Creator/12, Bus Creator1/1  "fix_type"
  Bus Selector/3 -> Data Type Conversion11/1  "<Sats>"
  Demux/1 -> latScale/1
  Demux/2 -> lonScale/1
  Demux/3 -> altScale/1
  ModelParam.GPSEphFinal/1 -> Gain1/1, Gain6/1
  Sum2/1 -> Motor_Dynamics_3/1
  Ve/1 -> VeScale1/1, Sum3/1
  GenCogVel/1(v) -> VelScale/1, VelScale1/1
  Eular(rad)/1 -> Selector/1
  Bus Creator/1 -> MavLinkGPS/1
  Bus Creator1/1 -> HILGPS/1
  -pi-pi---->0-2pi/1(yaw360) -> headVehAngleScale/1
  Selector/1 -> -pi-pi---->0-2pi/1(yaw180)
  BiasGain1/1 -> NoiseFilter1/1(In1)
  Uniform Random Number4/1 -> BiasGain1/1
  GenCogVel/2(cot) -> AngleScale/1, headMotAngle/1
  Sum1/1 -> Motor_Dynamics_1/1
  Uniform Random Number2/1 -> Sum1/2
  Uniform Random Number3/1 -> Sum2/2
  ModelParam.GPSEpvFinal/1 -> Gain8/1, Gain3/1
  Sum3/1 -> GenCogVel/1(u), VeScale/1
  NoiseFilter1/1(Out1) -> Sum3/2
  GPSFault/1 -> Bus Selector/1
  Xe1/1 -> GPSFault/1
  [FaultIn] -> GPSFault/2
  Bus Selector/1 -> Demux/1  "<GPSOut>"
  Bus Selector/2 -> Data Type Conversion10/1  "<3DFix>"

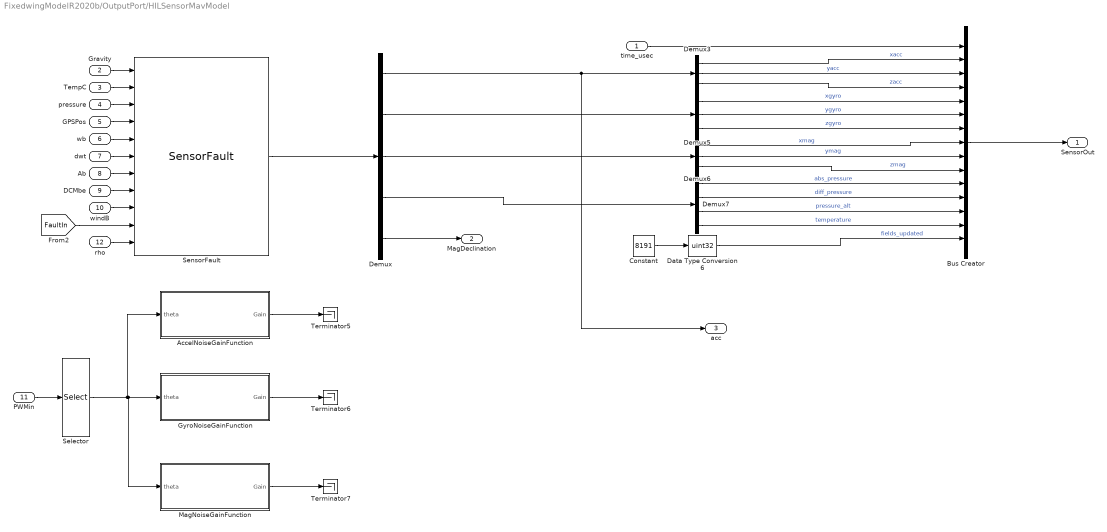
== system FixedwingModelR2020b/OutputPort/HILSensorMavModel ==
  time_usec : Inport
  Gravity : Inport  Port=2
  TempC : Inport  Port=3
  pressure : Inport  Port=4
  GPSPos : Inport  Port=5
  wb : Inport  Port=6
  dwt : Inport  Port=7
  Ab : Inport  Port=8
  DCMbe : Inport  Port=9
  windB : Inport  Port=10
  PWMin : Inport  Port=11
  rho : Inport  Port=12
  AccelNoiseGainFunction : MATLAB Function  TreatAsAtomicUnit=on
  Bus Creator : BusCreator  Inputs=15  OutDataTypeStr=Bus: MavLinkSensor  NonVirtualBus=on
  Constant : Constant  Value=8191
  Data Type Conversion6 : DataTypeConversion  OutDataTypeStr=uint32
  Demux : Demux  Outputs=5
  Demux3 : Demux  Outputs=3
  Demux5 : Demux  Outputs=3
  Demux6 : Demux  Outputs=3
  Demux7 : Demux
  GyroNoiseGainFunction : MATLAB Function  TreatAsAtomicUnit=on
  MagNoiseGainFunction : MATLAB Function  TreatAsAtomicUnit=on
  Selector : Selector  InputPortWidth=8  IndexOptions=Index vector (dialog)  Indices=[1]  OutputSizes=1
  SensorFault : FixedwingModelLib/SensorFault  FaultParamStruct=SensorFault  ComParamVect=FaultParamAPI
  Terminator5 : Terminator
  Terminator6 : Terminator
  Terminator7 : Terminator
  SensorOut : Outport  VectorParamsAs1DForOutWhenUnconnected=off
  MagDeclination : Outport  Port=2  VectorParamsAs1DForOutWhenUnconnected=off
  acc : Outport  Port=3  VectorParamsAs1DForOutWhenUnconnected=off
  wires:
  PWMin/1 -> Selector/1
  Demux7/4 -> Bus Creator/14  "temperature"
  Demux3/1 -> Bus Creator/2  "xacc"
  Demux6/3 -> Bus Creator/10  "zmag"
  time_usec/1 -> Bus Creator/1
  Demux3/3 -> Bus Creator/4  "zacc"
  Demux6/2 -> Bus Creator/9  "ymag"
  Demux6/1 -> Bus Creator/8  "xmag"
  Demux/5 -> MagDeclination/1
  Demux/1 -> acc/1, Demux3/1
  Demux7/2 -> Bus Creator/12  "diff_pressure"
  Demux7/3 -> Bus Creator/13  "pressure_alt"
  Demux5/2 -> Bus Creator/6  "ygyro"
  Demux7/1 -> Bus Creator/11  "abs_pressure"
  Demux5/1 -> Bus Creator/5  "xgyro"
  Demux3/2 -> Bus Creator/3  "yacc"
  SensorFault/1 -> Demux/1
  Data Type Conversion6/1 -> Bus Creator/15  "fields_updated"
  Demux/2 -> Demux5/1
  Bus Creator/1 -> SensorOut/1
  Demux/4 -> Demux7/1
  Constant/1 -> Data Type Conversion6/1
  Demux/3 -> Demux6/1
  Demux5/3 -> Bus Creator/7  "zgyro"
  TempC/1 -> SensorFault/2
  Gravity/1 -> SensorFault/1
  pressure/1 -> SensorFault/3
  GPSPos/1 -> SensorFault/4
  wb/1 -> SensorFault/5
  dwt/1 -> SensorFault/6
  Ab/1 -> SensorFault/7
  DCMbe/1 -> SensorFault/8
  windB/1 -> SensorFault/9
  rho/1 -> SensorFault/11
  [FaultIn] -> SensorFault/10
  Selector/1 -> AccelNoiseGainFunction/1(theta), MagNoiseGainFunction/1(theta), GyroNoiseGainFunction/1(theta)
  GyroNoiseGainFunction/1(Gain) -> Terminator6/1
  MagNoiseGainFunction/1(Gain) -> Terminator7/1
  AccelNoiseGainFunction/1(Gain) -> Terminator5/1

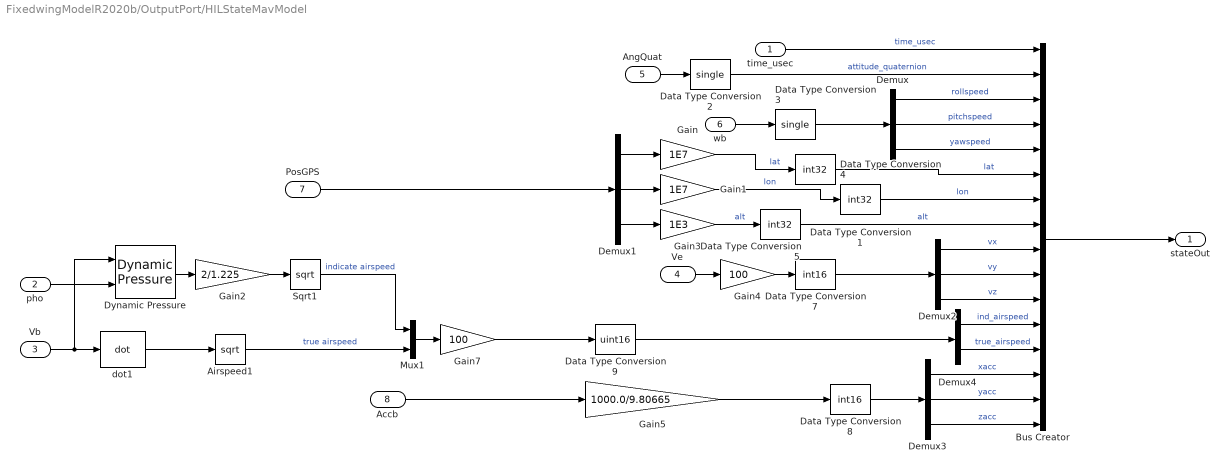
== system FixedwingModelR2020b/OutputPort/HILStateMavModel ==
  time_usec : Inport
  pho : Inport  Port=2
  Vb : Inport  Port=3
  Ve : Inport  Port=4
  AngQuat : Inport  Port=5
  wb : Inport  Port=6
  PosGPS : Inport  Port=7
  Accb : Inport  Port=8
  Airspeed1 : Sqrt  AlgorithmType=Newton-Raphson  SaturateOnIntegerOverflow=on
  Bus Creator : BusCreator  Inputs=16  OutDataTypeStr=Bus: MavLinkStateQuat  NonVirtualBus=on
  Data Type Conversion1 : DataTypeConversion  OutDataTypeStr=int32  RndMeth=Round
  Data Type Conversion2 : DataTypeConversion  OutDataTypeStr=single
  Data Type Conversion3 : DataTypeConversion  OutDataTypeStr=single
  Data Type Conversion4 : DataTypeConversion  OutDataTypeStr=int32  RndMeth=Round
  Data Type Conversion5 : DataTypeConversion  OutDataTypeStr=int32  RndMeth=Round
  Data Type Conversion7 : DataTypeConversion  OutDataTypeStr=int16  RndMeth=Round
  Data Type Conversion8 : DataTypeConversion  OutDataTypeStr=int16  RndMeth=Round
  Data Type Conversion9 : DataTypeConversion  OutDataTypeStr=uint16  RndMeth=Round
  Demux{,1..3} (4 alike) : Demux  Outputs=3
  Demux4 : Demux  Outputs=2
  Dynamic Pressure : aerolibasang/Dynamic Pressure
  Gain : Gain  Gain=1E7
  Gain1 : Gain  Gain=1E7
  Gain2 : Gain  Gain=2/1.225
  Gain3 : Gain  Gain=1E3
  Gain4 : Gain  Gain=100
  Gain5 : Gain  Gain=1000.0/9.80665
  Gain7 : Gain  Gain=100
  Mux1 : Mux  Inputs=2
  Sqrt1 : Sqrt  SaturateOnIntegerOverflow=on
  dot1 : aerolibasang/Incidence, Sideslip, & Airspeed/dot  SystemSampleTime=-1  VariantActivationTime=update diagram  Latency=0  AutoFrameSizeCalculation=off
      settings: SourceProductBaseCode=AE
  stateOut : Outport  VectorParamsAs1DForOutWhenUnconnected=off
  wires:
  Sqrt1/1 -> Mux1/1  "indicate airspeed"
  Gain2/1 -> Sqrt1/1
  Dynamic Pressure/1 -> Gain2/1
  time_usec/1 -> Bus Creator/1  "time_usec"
  Vb/1 -> dot1/1, Dynamic Pressure/1
  AngQuat/1 -> Data Type Conversion2/1
  Ve/1 -> Gain4/1
  wb/1 -> Data Type Conversion3/1
  Airspeed1/1 -> Mux1/2  "true airspeed"
  Mux1/1 -> Gain7/1
  Demux4/1 -> Bus Creator/12  "ind_airspeed"
  Demux4/2 -> Bus Creator/13  "true_airspeed"
  Demux3/3 -> Bus Creator/16  "zacc"
  Demux3/2 -> Bus Creator/15  "yacc"
  Demux3/1 -> Bus Creator/14  "xacc"
  Gain5/1 -> Data Type Conversion8/1
  Accb/1 -> Gain5/1
  Demux2/3 -> Bus Creator/11  "vz"
  Demux2/2 -> Bus Creator/10  "vy"
  Demux2/1 -> Bus Creator/9  "vx"
  Gain4/1 -> Data Type Conversion7/1
  Gain3/1 -> Data Type Conversion5/1  "alt"
  Gain1/1 -> Data Type Conversion1/1  "lon"
  Gain/1 -> Data Type Conversion4/1  "lat"
  Demux1/3 -> Gain3/1
  Demux1/2 -> Gain1/1
  Demux1/1 -> Gain/1
  Demux/3 -> Bus Creator/5  "yawspeed"
  Demux/2 -> Bus Creator/4  "pitchspeed"
  Demux/1 -> Bus Creator/3  "rollspeed"
  Data Type Conversion2/1 -> Bus Creator/2  "attitude_quaternion"
  pho/1 -> Dynamic Pressure/2
  Gain7/1 -> Data Type Conversion9/1
  dot1/1 -> Airspeed1/1
  Data Type Conversion3/1 -> Demux/1
  Data Type Conversion7/1 -> Demux2/1
  Data Type Conversion9/1 -> Demux4/1
  Data Type Conversion8/1 -> Demux3/1
  Data Type Conversion4/1 -> Bus Creator/6  "lat"
  Data Type Conversion1/1 -> Bus Creator/7  "lon"
  Data Type Conversion5/1 -> Bus Creator/8  "alt"
  Bus Creator/1 -> stateOut/1
  PosGPS/1 -> Demux1/1

== system FixedwingModelR2020b/OutputPort/To Sim Control ==
  Ve : Inport
  Xe : Inport  Port=2
  AngEuler : Inport  Port=3
  Rateb : Inport  Port=4
  Vb : Inport  Port=5
  Bus Creator : BusCreator  Inputs=16  OutDataTypeStr=Bus: StatesandOutput
      settings: InheritFromInputs=off
  Demux{,1..3,5} (5 alike) : Demux  Outputs=3
  States and Output : Outport  OutDataTypeStr=Bus: StatesandOutput  VectorParamsAs1DForOutWhenUnconnected=off
  wires:
  Bus Creator/1 -> States and Output/1
  Vb/1 -> Demux5/1
  Rateb/1 -> Demux3/1
  AngEuler/1 -> Demux2/1
  Xe/1 -> Demux1/1
  Ve/1 -> Demux/1
  [B] -> Bus Creator/16
  Demux5/3 -> Bus Creator/15  "W"
  Demux5/2 -> Bus Creator/14  "V"
  Demux5/1 -> Bus Creator/13  "U"
  Demux2/3 -> Bus Creator/9  "Psi"
  Demux2/2 -> Bus Creator/8  "The"
  Demux2/1 -> Bus Creator/7  "Phi"
  Demux3/3 -> Bus Creator/12  "R"
  Demux3/2 -> Bus Creator/11  "Q"
  Demux3/1 -> Bus Creator/10  "P"
  Demux1/3 -> Bus Creator/6  "Z"
  Demux1/2 -> Bus Creator/5  "Y"
  Demux1/1 -> Bus Creator/4  "X"
  Demux/3 -> Bus Creator/3  "Vz"
  Demux/2 -> Bus Creator/2  "Vy"
  Demux/1 -> Bus Creator/1  "Vx"

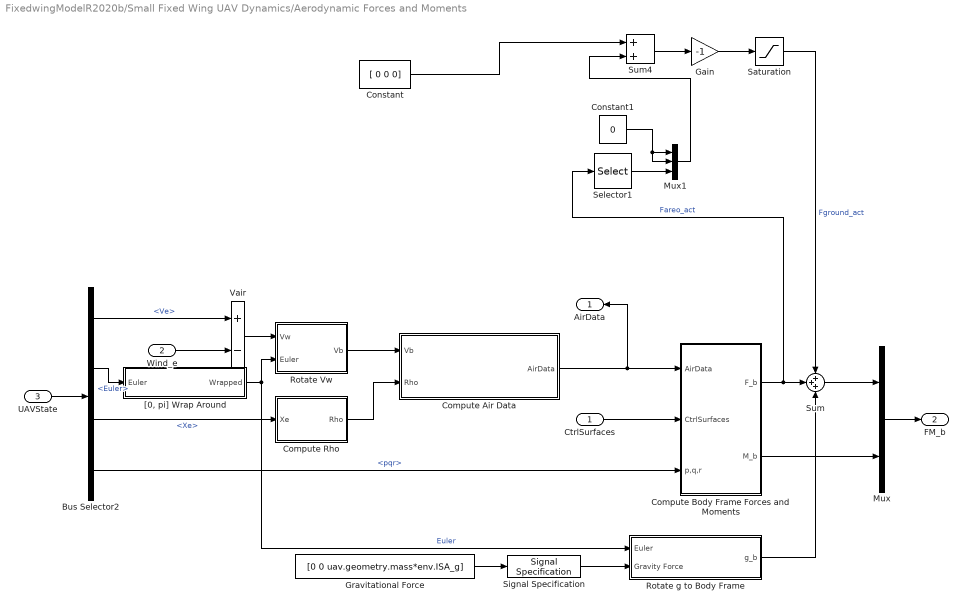
== system FixedwingModelR2020b/Small Fixed Wing UAV Dynamics/Aerodynamic Forces and Moments ==
  CtrlSurfaces : Inport
  Wind_e : Inport  Port=2
  UAVState : Inport  Port=3
  Bus Selector2 : BusSelector  OutputSignals=Ve,Euler,Xe,pqr
  Compute Air Data : Subsystem  TreatAsAtomicUnit=on  VariantControl=use_aerospace_blocks == 1
  Compute Body Frame Forces and Moments : Subsystem
  Compute Rho : Subsystem
  Constant : Constant  Value=[ 0 0 0]
      settings: AttributesFormatString=%<Value>
  Constant1 : Constant  Value=0
  Gain : Gain  Gain=-1
  Gravitational Force : Constant  Value=[0 0 uav.geometry.mass*env.ISA_g]  VectorParams1D=off
      settings: AttributesFormatString=%<Value>
  Mux : Mux  Inputs=2
  Mux1 : Mux  Inputs=3
  Rotate Vw : Subsystem
  Rotate g to Body Frame : Subsystem
  Saturation : Saturate  UpperLimit=0  LowerLimit=-inf
  Selector1 : Selector  InputPortWidth=3  IndexOptions=Index vector (dialog)  Indices=3  OutputSizes=1
  Signal Specification : SignalSpecification  Unit=kg*m/s^2
  Sum : Sum  Inputs=+++  SaturateOnIntegerOverflow=on
  Sum4 : Sum  InputSameDT=on  SaturateOnIntegerOverflow=on  OutDataTypeStr=Inherit: Same as first input
  Vair : Sum  Inputs=+-  InputSameDT=on  SaturateOnIntegerOverflow=on  OutDataTypeStr=Inherit: Same as first input
  "[0, pi] Wrap Around" : Subsystem
  AirData : Outport  VectorParamsAs1DForOutWhenUnconnected=off
  FM_b : Outport  Port=2  VectorParamsAs1DForOutWhenUnconnected=off
  wires:
  Bus Selector2/1 -> Vair/1  "<Ve>"
  UAVState/1 -> Bus Selector2/1
  Mux/1 -> FM_b/1
  Sum/1 -> Mux/1
  Wind_e/1 -> Vair/2
  CtrlSurfaces/1 -> Compute Body Frame Forces and Moments/2(CtrlSurfaces)
  Compute Air Data/1(AirData) -> AirData/1, Compute Body Frame Forces and Moments/1(AirData)
  Bus Selector2/4 -> Compute Body Frame Forces and Moments/3(p,q,r)  "<pqr>"
  Gravitational Force/1 -> Signal Specification/1
  Compute Body Frame Forces and Moments/2(M_b) -> Mux/2
  Rotate Vw/1(Vb) -> Compute Air Data/1(Vb)
  Compute Rho/1(Rho) -> Compute Air Data/2(Rho)
  Vair/1 -> Rotate Vw/1(Vw)
  Signal Specification/1 -> Rotate g to Body Frame/2(Gravity Force)
  Bus Selector2/3 -> Compute Rho/1(Xe)  "<Xe>"
  Saturation/1 -> Sum/1  "Fground_act"
  Gain/1 -> Saturation/1
  Constant/1 -> Sum4/1
  Constant1/1 -> Mux1/2, Mux1/1
  Mux1/1 -> Sum4/2
  Selector1/1 -> Mux1/3
  Sum4/1 -> Gain/1
  Compute Body Frame Forces and Moments/1(F_b) -> Sum/2, Selector1/1  "Fareo_act"
  Rotate g to Body Frame/1(g_b) -> Sum/3
  "[0, pi] Wrap Around"/1(Wrapped) -> Rotate g to Body Frame/1(Euler), Rotate Vw/2(Euler)  "Euler"
  Bus Selector2/2 -> "[0, pi] Wrap Around"/1(Euler)  "<Euler>"

== system FixedwingModelR2020b/Small Fixed Wing UAV Dynamics/Compute psi_dot ==
  Euler : Inport
  G : Inport  Port=2
  Mux1 : Mux  Inputs=2
  psidot : Fcn  Expr=(u[5]*sin(u[1])+u[6]*cos(u[1]))/cos(u[2])
  psi_dot : Outport  Unit=rad/S  VectorParamsAs1DForOutWhenUnconnected=off
  wires:
  G/1 -> Mux1/2
  psidot/1 -> psi_dot/1  "psi_dot"
  Mux1/1 -> psidot/1
  Euler/1 -> Mux1/1

== system FixedwingModelR2020b/Small Fixed Wing UAV Dynamics/GroundModel ==
  6DOF Bus : Inport
  "tZ " : Inport  Port=2
  Bus Selector : BusSelector  OutputSignals=Xe,Ve,Eular(rad),DCM,wb
  Direction Cosine Matrix to Quaternions : sharedtransform/Direction Cosine Matrix  to Quaternions  aMode=aMode  action=None  tolerance=eps(2)
      settings: SourceProductBaseCode=AE,PW,DR,MT,VE
  Direction Cosine Matrix to Quaternions1 : sharedtransform/Direction Cosine Matrix  to Quaternions  aMode=aMode  action=None  tolerance=eps(2)
      settings: SourceProductBaseCode=AE,PW,DR,MT,VE
  Euler to DCM : aerolibtransform2/Wind Angles to  Direction Cosine Matrix
      settings: SourceProductBaseCode=AE
  Gain : Gain  Gain=[0 0 9.8]
  Ground Model : MATLAB Function  TreatAsAtomicUnit=on
  ModelParam.uavMass : Constant  Value=uav.geometry.mass
  Mux : Mux  Inputs=2
  OnGroundFaceup : MATLAB Function  TreatAsAtomicUnit=on
  Product : Product  Multiplication=Matrix(*)
  Quaternion Inverse : aerolibutil/Quaternion Inverse
  Quaternion Multiplication : aerolibutil/Quaternion Multiplication
  Terminator : Terminator
  Terminator1 : Terminator
  FM : Outport  VectorParamsAs1DForOutWhenUnconnected=off
  wires:
  Ground Model/4(takeoff) -> Terminator/1
  "tZ "/1 -> Ground Model/6(terrainZ)
  Ground Model/2(M1) -> Mux/2  "Mb"
  Product/1 -> Mux/1  "Fb"
  Quaternion Multiplication/1 -> Ground Model/5(Quet)
  Quaternion Inverse/1 -> Quaternion Multiplication/1
  Direction Cosine Matrix to Quaternions1/1 -> Quaternion Inverse/1
  Euler to DCM/1 -> Direction Cosine Matrix to Quaternions1/1
  OnGroundFaceup/1(y) -> Euler to DCM/1
  Direction Cosine Matrix to Quaternions/1 -> Quaternion Multiplication/2
  Ground Model/1(F1) -> Product/2
  Bus Selector/4 -> Direction Cosine Matrix to Quaternions/1, Product/1  "<DCM>"
  Bus Selector/5 -> Ground Model/2(wb)  "<wb>"
  6DOF Bus/1 -> Bus Selector/1
  Bus Selector/2 -> Ground Model/4(Ve)  "<Ve>"
  Bus Selector/1 -> Ground Model/3(Xe)  "<Xe>"
  Bus Selector/3 -> OnGroundFaceup/1(EulerAng)  "<Eular(rad)>"
  Ground Model/3(landed) -> Terminator1/1  "landed"
  Mux/1 -> FM/1
  ModelParam.uavMass/1 -> Gain/1
  Gain/1 -> Ground Model/1(mg)

== system FixedwingModelR2020b/Weather Model/ Compute Norm ==
  <Ve> : Inport
  Dot Product : DotProduct  InputSameDT=on  OutDataTypeStr=Inherit: Inherit via internal rule
  Math Function1 : Sqrt  AlgorithmType=Newton-Raphson  SaturateOnIntegerOverflow=on
      settings: AttributesFormatString=%<AlgorithmType>
  Zero Bound : Saturate  UpperLimit=inf  LowerLimit=0.001
      settings: AttributesFormatString="[%<LowerLimit>  %<UpperLimit>]"
  V : Outport  VectorParamsAs1DForOutWhenUnconnected=off
  wires:
  Dot Product/1 -> Zero Bound/1
  Zero Bound/1 -> Math Function1/1
  <Ve>/1 -> Dot Product/2, Dot Product/1
  Math Function1/1 -> V/1

== system FixedwingModelR2020b/Weather Model/RL2B ==
  Euler : Inport
  Rotation Angles to Direction Cosine Matrix : sharedtransform/Rotation Angles to Direction Cosine Matrix  rotationOrder=ZYX  aMode=aMode
      settings: SourceProductBaseCode=AE,PW,DR,MT,VE
  Selector : Selector  InputPortWidth=3  IndexOptions=Index vector (dialog)  Indices=[3 2 1]  OutputSizes=1
  RL2B : Outport  VectorParamsAs1DForOutWhenUnconnected=off
  wires:
  Rotation Angles to Direction Cosine Matrix/1 -> RL2B/1
  Euler/1 -> Selector/1
  Selector/1 -> Rotation Angles to Direction Cosine Matrix/1

== system FixedwingModelR2020b/Weather Model/[0, pi] Wrap Around ==
  Euler : Inport
  Compare To Zero : simulink/Logic and Bit Operations/Compare To Zero  relop=>=  OutDataTypeStr=uint8  ZeroCross=off
  Logical Operator : Logic  Operator=NOT  AllPortsSameDT=off  OutDataTypeStr=boolean
  Merge : Merge  InitialOutput=0
  Mux2 : Mux  Inputs=2
  Negative Yaw : Subsystem
  Positive Yaw : Subsystem
  Selector1 : Selector  InputPortWidth=3  IndexOptions=Index vector (dialog)  Indices=[1 2]  OutputSizes=1
  Selector2 : Selector  InputPortWidth=3  IndexOptions=Index vector (dialog)  Indices=[3]  OutputSizes=1
  Wrapped : Outport  VectorParamsAs1DForOutWhenUnconnected=off
  wires:
  Negative Yaw/1(yaw_wr) -> Merge/2
  Positive Yaw/1(yaw_wr) -> Merge/1
  Merge/1 -> Mux2/2
  Logical Operator/1 -> Negative Yaw/Enable
  Compare To Zero/1 -> Logical Operator/1, Positive Yaw/Enable
  Selector2/1 -> Negative Yaw/1(yaw), Positive Yaw/1(yaw), Compare To Zero/1
  Mux2/1 -> Wrapped/1
  Selector1/1 -> Mux2/1
  Euler/1 -> Selector1/1, Selector2/1

== system FixedwingModelR2020b/Motor Model/Engine Model/Get To ==
  dt : Inport
  Divide : Product  Inputs=3
  Math Function : Math  Operator=pow  SignedPower=on  SaturateOnIntegerOverflow=on
  Math Function1 : Math  Operator=pow  SignedPower=on  SaturateOnIntegerOverflow=on
  MaxRPM : Gain  Gain=8000  SaturateOnIntegerOverflow=on  OutDataTypeStr=Inherit: Same as input  ParamDataTypeStr=Inherit: Same as input
      settings: AttributesFormatString=%<Gain>
  MaxRPM1 : Gain  Gain=uav.engine.TFact  SaturateOnIntegerOverflow=on  OutDataTypeStr=Inherit: Same as input  ParamDataTypeStr=Inherit: Same as input
      settings: AttributesFormatString=%<Gain>
  Min RPM : Constant  Value=0
      settings: AttributesFormatString=%<Value>
  Min Th K : Constant  Value=uav.engine.MinThK
      settings: AttributesFormatString=%<Value>
  Prop Diameter (in) : Constant  Value=17
      settings: AttributesFormatString=%<Value>
  Prop Diameter (in)1 : Constant  Value=2
      settings: AttributesFormatString=%<Value>
  Prop Diameter (in)2 : Constant  Value=4
      settings: AttributesFormatString=%<Value>
  Saturation : Saturate  UpperLimit=1.0  LowerLimit=0
      settings: AttributesFormatString="[%<LowerLimit>  %<UpperLimit>]"
  Sum : Sum  Inputs=|++
  Sum1 : Sum  Inputs=|++
  Th K : Gain  Gain=uav.engine.ThK  SaturateOnIntegerOverflow=on  OutDataTypeStr=Inherit: Same as input  ParamDataTypeStr=Inherit: Same as input
      settings: AttributesFormatString=%<Gain>
  To Constant : Constant  Value=2.83e-12
      settings: AttributesFormatString=%<Value>
  To : Outport  VectorParamsAs1DForOutWhenUnconnected=off
  wires:
  Min Th K/1 -> Sum1/2
  Sum1/1 -> MaxRPM/1
  dt/1 -> Saturation/1
  Th K/1 -> Sum1/1
  MaxRPM/1 -> Sum/1
  Min RPM/1 -> Sum/2
  Sum/1 -> Math Function/1
  MaxRPM1/1 -> To/1
  Divide/1 -> MaxRPM1/1
  To Constant/1 -> Divide/3
  Math Function1/1 -> Divide/2
  Math Function/1 -> Divide/1
  Prop Diameter (in)/1 -> Math Function1/1
  Prop Diameter (in)2/1 -> Math Function1/2
  Prop Diameter (in)1/1 -> Math Function/2
  Saturation/1 -> Th K/1
